simulink model "two_DF_unsplant1"  (Simulink 7.9)
settings: Solver=ode4  SolverMode=SingleTasking  StartTime=0.0  StopTime=120.0  FixedStep=Tm  RelTol=1e-3
InitFcn:
  | initcond
values from neighbouring files (symbols this model uses):
  Delay = 0.5    [initcond.m]    (also in initcond_2DOF_unsplant1.m; initcond_2DOF_unsplant1_copy.m)
  Tm = 0.01    [initcond.m]    (also in initcond_2DOF_unsplant1.m; initcond_2DOF_unsplant1_copy.m)
libraries: fuzblock x3
settings Model: Creator=Ponciano Jorge  LastModifiedBy=cic-pjea  ExtModeTrigMode=oneshot  ExtModeArmWhenConnect=off
settings DataIOCC: LimitDataPoints=off
settings OptimizationCC: BlockReduction=off  BooleanDataType=off  InitFltsAndDblsToZero=on
settings DebuggingCC: SaveWithParameterizedLinksMsg=none  SignalResolutionControl=TryResolveAllWithWarning  SolverPrmCheckMsg=none  MultiTaskDSMMsg=warning  MultiTaskCondExecSysMsg=none  FcnCallInpInsideContextMsg=Use local settings  StrictBusMsg=None
settings HardwareCC: TargetUnknown=on
settings RTWCC: IncludeERTFirstTime=on
settings GRTTargetCC: CombineOutputUpdateFcns=off  GRTInterface=on

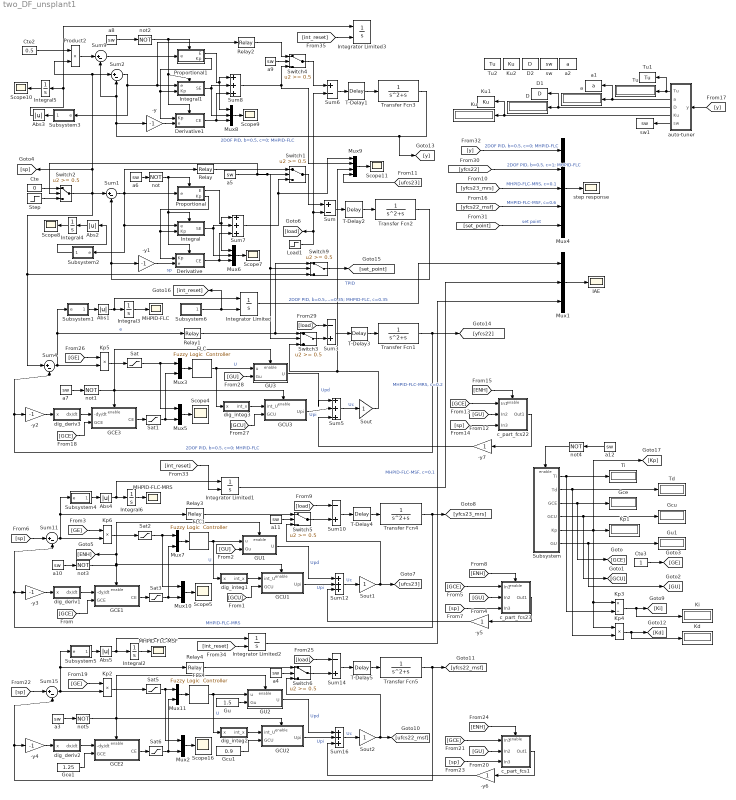
== system two_DF_unsplant1 ==
  -y{,1..4} (5 alike) : Gain  Gain=-1  SaturateOnIntegerOverflow=on  OutDataTypeStr=Inherit: Same as input  ParamDataTypeStr=Inherit: Same as input
  -y5 : Gain  SaturateOnIntegerOverflow=on  OutDataTypeStr=Inherit: Same as input  ParamDataTypeStr=Inherit: Same as input
  -y6 : Gain  SaturateOnIntegerOverflow=on  OutDataTypeStr=Inherit: Same as input  ParamDataTypeStr=Inherit: Same as input
  -y7 : Gain  SaturateOnIntegerOverflow=on  OutDataTypeStr=Inherit: Same as input  ParamDataTypeStr=Inherit: Same as input
  Abs{1..5} (5 alike) : Abs  SaturateOnIntegerOverflow=on
  Cte : Constant  Value=0
  Cte2 : Constant  Value=0.5
  Cte3 : Constant
  D : Display
  D1 : DataStoreWrite  DataStoreName=D
  D2 : DataStoreMemory  DataStoreName=D
  Derivative : Subsystem  TreatAsAtomicUnit=on
  Derivative1 : Subsystem  TreatAsAtomicUnit=on
  FLC : fuzblock/Fuzzy Logic  Controller  fis=stfc22
  FLC1 : fuzblock/Fuzzy Logic  Controller  fis=fcs_unsplan1
  FLC4 : fuzblock/Fuzzy Logic  Controller  fis=stfc22
  GCE1 : Subsystem  TreatAsAtomicUnit=on
  GCE2 : Subsystem  TreatAsAtomicUnit=on
  GCE3 : Subsystem  TreatAsAtomicUnit=on
  GCU1 : Subsystem  TreatAsAtomicUnit=on
  GCU2 : Subsystem  TreatAsAtomicUnit=on
  GCU3 : Subsystem  TreatAsAtomicUnit=on
  GU1 : Subsystem  TreatAsAtomicUnit=on
  GU2 : Subsystem  TreatAsAtomicUnit=on
  GU3 : Subsystem  TreatAsAtomicUnit=on
  Gce : Display
  Gce1 : Constant  Value=1.25
  Gcu : Display
  Gcu1 : Constant  Value=0.9
  Gu : Constant  Value=1.5
  Gu1 : Display
  IAE : Scope
      settings: TickLabels=on  ShowLegends=on  TimeRange=60.03765050579885  YMin=0  YMax=3.5  SaveName=G
  Integral : Subsystem  TreatAsAtomicUnit=on
  Integral1 : Subsystem  TreatAsAtomicUnit=on
  Integral{2..6} (5 alike) : TransferFcn  Denominator=[1 0]
  Integrator Limited{,1..3} (4 alike) : Integrator  ExternalReset=rising  UpperSaturationLimit=1  LowerSaturationLimit=0
  Kd : Display
  Ki : Display
  Kp1 : Display
  Kp2 : Product  SaturateOnIntegerOverflow=on  RndMeth=Zero  InputSameDT=on  OutDataTypeStr=Inherit: Same as first input
  Kp3 : Product  Inputs=*/  SaturateOnIntegerOverflow=on  RndMeth=Zero  InputSameDT=on  OutDataTypeStr=Inherit: Same as first input
  Kp4 : Product  Inputs=**  SaturateOnIntegerOverflow=on  RndMeth=Zero  InputSameDT=on  OutDataTypeStr=Inherit: Same as first input
  Kp5 : Product  SaturateOnIntegerOverflow=on  RndMeth=Zero  InputSameDT=on  OutDataTypeStr=Inherit: Same as first input
  Kp6 : Product  SaturateOnIntegerOverflow=on  RndMeth=Zero  InputSameDT=on  OutDataTypeStr=Inherit: Same as first input
  Ku : Display
  Ku1 : DataStoreWrite  DataStoreName=Ku
  Ku2 : DataStoreMemory  DataStoreName=Ku
  Load1 : Step  Time=92  SampleTime=0
  MHPID-FLC : Scope
      settings: TimeRange=120  YMin=0  YMax=6
  MHPID-FLC-MRS : Scope
      settings: TimeRange=25.06031417248357  YMin=0  YMax=2  SaveName=ScopeData3
  MHPID-FLC-MSF : Scope
      settings: TimeRange=25.04235461740161  YMin=0  YMax=2  SaveName=ScopeData6
  Mux1 : Mux  Inputs=3
  Mux{2..3,5,7,10..11} (6 alike) : Mux  Inputs=2
  Mux4 : Mux  Inputs=5
  Mux6 : Mux  Inputs=3
  Mux8 : Mux  Inputs=3
  Mux9 : Mux
  Product2 : Product  Inputs=**  SaturateOnIntegerOverflow=on  RndMeth=Zero  InputSameDT=on  OutDataTypeStr=Inherit: Same as first input
  Proportional : Subsystem  TreatAsAtomicUnit=on
  Proportional1 : Subsystem  TreatAsAtomicUnit=on
  Relay{,1..4} (5 alike) : Relay  OnOutputValue=0.1  OffOutputValue=-0.1
  Sat{,1..3,5..6} (6 alike) : Saturate  UpperLimit=1  LowerLimit=-1
  Scope{4..5,7..11,16} (8 alike) : Scope
      Scope10 settings: TimeRange=120  YMin=0  YMax=6
      Scope11 settings: TimeRange=50  YMin=-1
      Scope16 settings: TimeRange=40  YMin=-1  YMax=1  SaveName=ScopeData5
      Scope4 settings: TimeRange=50  YMin=-1  YMax=1
      Scope5 settings: TimeRange=40  YMin=-1  YMax=1  SaveName=ScopeData4
      Scope7 settings: TimeRange=50  YMin=-2  YMax=4
      Scope8 settings: TimeRange=120  YMin=0  YMax=7
      Scope9 settings: TimeRange=50  YMin=-2.71141  YMax=4
  Sout : Gain  SaturateOnIntegerOverflow=on  OutDataTypeStr=Inherit: Same as input  ParamDataTypeStr=Inherit: Same as input
  Sout1 : Gain  SaturateOnIntegerOverflow=on  OutDataTypeStr=Inherit: Same as input  ParamDataTypeStr=Inherit: Same as input
  Sout2 : Gain  SaturateOnIntegerOverflow=on  OutDataTypeStr=Inherit: Same as input  ParamDataTypeStr=Inherit: Same as input
  Step : Step  Time=65  SampleTime=0
  Subsystem : Subsystem  TreatAsAtomicUnit=on
  Subsystem1 : Subsystem
  Subsystem2 : Subsystem
  Subsystem3 : Subsystem
  Subsystem4 : Subsystem
  Subsystem5 : Subsystem
  Subsystem6 : Subsystem
  Sum : Sum  Inputs=+-  SaturateOnIntegerOverflow=on  InputSameDT=on  OutDataTypeStr=Inherit: Same as first input
  Sum{1..2,4,9,11,15} (6 alike) : Sum  Inputs=|+-  SaturateOnIntegerOverflow=on  InputSameDT=on  OutDataTypeStr=Inherit: Same as first input
  Sum10 : Sum  Inputs=-+  SaturateOnIntegerOverflow=on  InputSameDT=on  OutDataTypeStr=Inherit: Same as first input
  Sum12 : Sum  Inputs=+++  SaturateOnIntegerOverflow=on  InputSameDT=on  OutDataTypeStr=Inherit: Same as first input
  Sum14 : Sum  Inputs=-+  SaturateOnIntegerOverflow=on  InputSameDT=on  OutDataTypeStr=Inherit: Same as first input
  Sum16 : Sum  Inputs=+++  SaturateOnIntegerOverflow=on  InputSameDT=on  OutDataTypeStr=Inherit: Same as first input
  Sum3 : Sum  Inputs=-+  SaturateOnIntegerOverflow=on  InputSameDT=on  OutDataTypeStr=Inherit: Same as first input
  Sum5 : Sum  Inputs=|+++  SaturateOnIntegerOverflow=on  InputSameDT=on  OutDataTypeStr=Inherit: Same as first input
  Sum6 : Sum  Inputs=+-  SaturateOnIntegerOverflow=on  InputSameDT=on  OutDataTypeStr=Inherit: Same as first input
  Sum7 : Sum  Inputs=|+++  SaturateOnIntegerOverflow=on  InputSameDT=on  OutDataTypeStr=Inherit: Same as first input
  Sum8 : Sum  Inputs=|+++  SaturateOnIntegerOverflow=on  InputSameDT=on  OutDataTypeStr=Inherit: Same as first input
  Switch{1..6,9} (7 alike) : Switch  Threshold=0.5  SaturateOnIntegerOverflow=on  InputSameDT=on
  T-Delay{1..5} (5 alike) : TransportDelay  DelayTime=Delay
  Td : Display
  Ti : Display
  Transfer Fcn{1..5} (5 alike) : TransferFcn  Denominator=[1 1 0]
  Tu : Display
  Tu1 : DataStoreWrite  DataStoreName=Tu
  Tu2 : DataStoreMemory  DataStoreName=Tu  InitialValue=1
  a : Display
  a1 : DataStoreWrite  DataStoreName=a
  a{3..12} (10 alike) : DataStoreRead  DataStoreName=sw  SampleTime=0
  a2 : DataStoreMemory  DataStoreName=a
  auto-tuner : Subsystem
  c_part_fcs1 : Subsystem
  c_part_fcs22 : Subsystem
  c_part_fcs23 : Subsystem
  dig_deriv1 : Subsystem
  dig_deriv2 : Subsystem
  dig_deriv3 : Subsystem
  dig_integ1 : Subsystem
  dig_integ2 : Subsystem
  dig_integ3 : Subsystem
  not{,1..5} (6 alike) : Logic  Operator=NOT
  step response : Scope
      settings: TickLabels=on  ShowLegends=on  TimeRange=60.03765050579885  YMin=-0.2  YMax=1.4  SaveName=G3
  sw : DataStoreMemory  DataStoreName=sw
  sw1 : DataStoreWrite  DataStoreName=sw
  wires:
  T-Delay2/1 -> Transfer Fcn2/1
  Mux3/1 -> FLC/1
  T-Delay3/1 -> Transfer Fcn1/1
  Step/1 -> Switch2/3
  Cte/1 -> Switch2/1
  Transfer Fcn1/1 -> [yfcs22], Sum4/2, -y2/1  "2DOF PID, b=0.5, c=0; MHPID-FLC"
  Sum1/1 -> Proportional/1(e), Integral/1(e), Subsystem2/1(e), Relay/1
  Sum5/1 -> Sout/1  "Uc"
  a6/1 -> not/1
  not/1 -> Proportional/Enable, Integral/Enable, Derivative/Enable
  Proportional/2(Kp) -> Derivative/1(Kp), Integral/2(Kp)
  a7/1 -> not1/1
  Mux5/1 -> Scope4/1
  not1/1 -> GU3/Enable, GCE3/Enable, GCU3/Enable
  Switch2/1 -> Switch9/3, Sum4/1, Sum1/1, Sum2/1, Product2/2, [sp]  "sp"
  Load1/1 -> Sum6/2, Sum/2, [load]
  auto-tuner/1(Tu) -> Tu/1, Tu1/1
  auto-tuner/2(a) -> a/1, a1/1
  auto-tuner/3(D) -> D/1, D1/1
  auto-tuner/4(Ku) -> Ku/1, Ku1/1
  auto-tuner/5(sw) -> sw1/1
  Subsystem1/1(Out1) -> Abs1/1
  Abs1/1 -> Integral3/1, Integrator Limited/1
  Integral3/1 -> MHPID-FLC/1
  Integral4/1 -> Scope8/1
  Abs2/1 -> Integral4/1
  Subsystem2/1(Out1) -> Abs2/1
  Proportional1/2(Kp) -> Derivative1/1(Kp), Integral1/2(Kp)
  a8/1 -> not2/1
  not2/1 -> Proportional1/Enable, Derivative1/Enable, Integral1/Enable
  T-Delay1/1 -> Transfer Fcn3/1
  Product2/1 -> Sum9/1
  Sum2/1 -> Integral1/1(e), Relay2/1, Subsystem3/1(e)
  Sum9/1 -> Proportional1/1(e)
  a5/1 -> Switch1/2, Switch2/2, Switch3/2, Switch9/2
  Mux6/1 -> Scope7/1
  Derivative/1(CE) -> Sum7/3, Mux6/3
  Mux8/1 -> Scope9/1
  Derivative1/1(CE) -> Sum8/3, Mux8/3
  Integral1/1(SE) -> Sum8/2, Mux8/2
  Proportional1/1(E) -> Sum8/1, Mux8/1
  Integral/1(SE) -> Sum7/2, Mux6/2
  Proportional/1(E) -> Sum7/1, Mux6/1
  a9/1 -> Switch4/2
  Relay2/1 -> Switch4/1
  Switch4/1 -> Sum6/1
  Sum4/1 -> Relay1/1, Subsystem1/1(e), Kp5/2  "e"
  Relay/1 -> Switch1/1
  Relay1/1 -> Switch3/1, Switch9/1
  Integral5/1 -> Scope10/1
  Subsystem3/1(Out1) -> Abs3/1
  Abs3/1 -> Integral5/1, Integrator Limited3/1
  Mux9/1 -> Scope11/1
  Sum6/1 -> T-Delay1/1
  Sum/1 -> T-Delay2/1
  Sum3/1 -> T-Delay3/1
  Sum8/1 -> Switch4/3, Mux9/2
  Subsystem/1(Ti) -> Ti/1, Kp3/2
  Subsystem/3(GCE) -> Gce/1, [GCE]
  Subsystem/5(Kp) -> Kp1/1, Kp3/1, Kp4/1, [Kp]
  a12/1 -> not4/1
  not4/1 -> Subsystem/Enable
  Subsystem/2(Td) -> Td/1, Kp4/2
  Subsystem/6(GU) -> Gu1/1, [GU]
  Transfer Fcn3/1 -> Sum2/2, Sum9/2, -y/1, [y]  "2DOF PID, b=0.5, c=0; MHPID-FLC"
  Transfer Fcn2/1 -> Sum1/2, -y1/1  "TPID"
  Switch1/1 -> Sum/1
  Sum7/1 -> Switch1/3, Mux9/1
  Subsystem/4(GCU) -> Gcu/1, [GCU]
  Sat/1 -> Mux3/1, Mux5/1
  Sat1/1 -> Mux3/2, Mux5/2
  GCE3/1(CE) -> Sat1/1
  Switch3/1 -> Sum3/2
  Sout/1 -> Switch3/3, Mux9/3
  dig_deriv3/1(dx/dt) -> GCE3/1(-dy/dt)
  dig_integ3/1(int_x) -> GCU3/1(int_U)
  GCU3/1(Upi) -> Sum5/2  "Upi"
  GU3/1(U) -> Sum5/1  "Upd"
  -y1/1 -> Derivative/2(e)
  -y2/1 -> dig_deriv3/1(x)
  FLC/1 -> dig_integ3/1(x), GU3/1(u)  "U"
  -y/1 -> Derivative1/2(e)
  Cte2/1 -> Product2/1
  Cte3/1 -> [GE]
  [ufcs23] -> Mux9/4
  [GCE] -> c_part_fcs22/1(In1)
  [sp] -> c_part_fcs22/3(In3)
  [GU] -> c_part_fcs22/2(In2)
  [ENH] -> c_part_fcs22/Enable
  Mux7/1 -> FLC1/1
  GCU1/1(Upi) -> Sum12/2  "Upi"
  T-Delay4/1 -> Transfer Fcn4/1
  Sum12/1 -> Sout1/1  "Uc"
  a10/1 -> not3/1
  dig_deriv1/1(dx/dt) -> GCE1/1(-dy/dt)
  Mux10/1 -> Scope5/1
  FLC1/1 -> GU1/1(u), dig_integ1/1(x)  "U"
  GU1/1(U) -> Sum12/1  "Upd"
  Subsystem4/1(Out1) -> Abs4/1
  Abs4/1 -> Integral6/1, Integrator Limited1/1
  Integral6/1 -> MHPID-FLC-MRS/1
  Sum11/1 -> Relay3/1, Subsystem4/1(e), Kp6/2
  Switch5/1 -> Sum10/2
  Sum10/1 -> T-Delay4/1
  GCE1/1(CE) -> Sat3/1
  Sat3/1 -> Mux7/2, Mux10/2
  Kp6/1 -> Sat2/1
  Sat2/1 -> Mux7/1, Mux10/1
  Relay3/1 -> Switch5/1
  a11/1 -> Switch5/2
  Transfer Fcn4/1 -> -y3/1, Sum11/2, [yfcs23_mrs]  "MHPID-FLC-MRS"
  Sout1/1 -> Switch5/3, [ufcs23]
  -y3/1 -> dig_deriv1/1(x)
  [GCE] -> GCE1/2(GCE)
  [GE] -> Kp6/1
  dig_integ1/1(int_x) -> GCU1/1(int_U)
  [GCU] -> GCU1/2(GCU)
  [GU] -> GU1/2(Gu)
  not3/1 -> GCE1/Enable, GCU1/Enable, GU1/Enable, [ENH]
  [GU] -> c_part_fcs23/2(In2)
  [GCE] -> c_part_fcs23/1(In1)
  [sp] -> Sum11/1
  [sp] -> c_part_fcs23/3(In3)
  [ENH] -> c_part_fcs23/Enable
  c_part_fcs23/1(Out1) -> -y5/1
  [load] -> Sum10/1
  Mux11/1 -> FLC4/1
  GCU2/1(Upi) -> Sum16/2  "Upi"
  T-Delay5/1 -> Transfer Fcn5/1
  Sum16/1 -> Sout2/1  "Uc"
  a3/1 -> not5/1
  dig_deriv2/1(dx/dt) -> GCE2/1(-dy/dt)
  Mux2/1 -> Scope16/1
  FLC4/1 -> GU2/1(u), dig_integ2/1(x)  "U"
  GU2/1(U) -> Sum16/1  "Upd"
  Subsystem5/1(Out1) -> Abs5/1
  Abs5/1 -> Integral2/1, Integrator Limited2/1
  Integral2/1 -> MHPID-FLC-MSF/1
  Sum15/1 -> Relay4/1, Subsystem5/1(e), Kp2/2
  Switch6/1 -> Sum14/2
  Sum14/1 -> T-Delay5/1
  GCE2/1(CE) -> Sat6/1
  Sat6/1 -> Mux11/2, Mux2/2
  Kp2/1 -> Sat5/1
  Sat5/1 -> Mux11/1, Mux2/1
  Relay4/1 -> Switch6/1
  a4/1 -> Switch6/2
  Transfer Fcn5/1 -> -y4/1, Sum15/2, [yfcs22_msf]
  Sout2/1 -> Switch6/3, [ufcs22_msf]
  -y4/1 -> dig_deriv2/1(x)
  [GE] -> Kp2/1
  dig_integ2/1(int_x) -> GCU2/1(int_U)
  not5/1 -> GCE2/Enable, GU2/Enable, GCU2/Enable
  [GU] -> c_part_fcs1/2(In2)
  [GCE] -> c_part_fcs1/1(In1)
  [sp] -> Sum15/1
  [sp] -> c_part_fcs1/3(In3)
  [ENH] -> c_part_fcs1/Enable
  [load] -> Sum14/1
  Kp3/1 -> [Ki], Ki/1
  Kp4/1 -> [Kd], Kd/1
  Gu/1 -> GU2/2(Gu)
  Gcu1/1 -> GCU2/2(GCU)
  Gce1/1 -> GCE2/2(GCE)
  c_part_fcs1/1(Out1) -> -y6/1
  -y5/1 -> Sum12/3
  -y6/1 -> Sum16/3
  -y7/1 -> Sum5/3
  Mux1/1 -> IAE/1
  Subsystem6/1(Out1) -> Integrator Limited/2, [int_reset]
  [int_reset] -> Integrator Limited1/2
  Integrator Limited1/1 -> Mux1/2  "MHPID-FLC-MRS, c=0.2"
  [int_reset] -> Integrator Limited2/2
  Integrator Limited2/1 -> Mux1/3  "MHPID-FLC-MSF, c=0.1"
  [y] -> auto-tuner/1(y)
  [GCE] -> GCE3/2(GCE)
  [GE] -> Kp5/1
  Kp5/1 -> Sat/1
  [GCU] -> GCU3/2(GCU)
  [GU] -> GU3/2(Gu)
  [load] -> Sum3/1
  c_part_fcs22/1(Out1) -> -y7/1
  Switch9/1 -> [set_point]
  Mux4/1 -> step response/1
  [int_reset] -> Integrator Limited3/2
  Integrator Limited/1 -> Mux1/1  "2DOF PID, b=0.5, c=0.35; MHPID-FLC, c=0.35"
  [y] -> Mux4/1  "2DOF PID, b=0.5, c=0; MHPID-FLC"
  [yfcs22] -> Mux4/2  "2DOF PID, b=0.5, c=1; MHPID-FLC"
  [yfcs23_mrs] -> Mux4/3  "MHPID-FLC-MRS, c=0.1"
  [yfcs22_msf] -> Mux4/4  "MHPID-FLC-MSF, c=0.6"
  [set_point] -> Mux4/5  "set point"

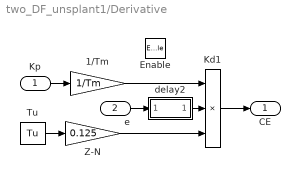
== system two_DF_unsplant1/Derivative ==
  Kp : Inport
  e : Inport  Port=2
  Enable : EnablePort
  1/Tm : Gain  Gain=1/Tm  SaturateOnIntegerOverflow=on  OutDataTypeStr=Inherit: Same as input  ParamDataTypeStr=Inherit: Same as input
  Kd1 : Product  Inputs=3  SaturateOnIntegerOverflow=on  RndMeth=Zero  InputSameDT=on  OutDataTypeStr=Inherit: Same as first input
  Tu : DataStoreRead  DataStoreName=Tu  SampleTime=0
  Z-N : Gain  Gain=0.125  SaturateOnIntegerOverflow=on  OutDataTypeStr=Inherit: Same as input  ParamDataTypeStr=Inherit: Same as input
  delay2 : Subsystem
  CE : Outport
  wires:
  e/1 -> delay2/1(In1)
  Kd1/1 -> CE/1
  Tu/1 -> Z-N/1
  Z-N/1 -> Kd1/3
  Kp/1 -> 1/Tm/1
  1/Tm/1 -> Kd1/1
  delay2/1(Out1) -> Kd1/2

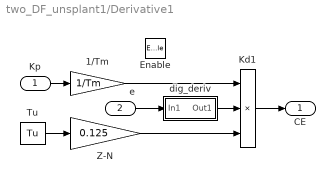
== system two_DF_unsplant1/Derivative1 ==
  Kp : Inport
  e : Inport  Port=2
  Enable : EnablePort
  1/Tm : Gain  Gain=1/Tm  SaturateOnIntegerOverflow=on  OutDataTypeStr=Inherit: Same as input  ParamDataTypeStr=Inherit: Same as input
  Kd1 : Product  Inputs=3  SaturateOnIntegerOverflow=on  RndMeth=Zero  InputSameDT=on  OutDataTypeStr=Inherit: Same as first input
  Tu : DataStoreRead  DataStoreName=Tu  SampleTime=0
  Z-N : Gain  Gain=0.125  SaturateOnIntegerOverflow=on  OutDataTypeStr=Inherit: Same as input  ParamDataTypeStr=Inherit: Same as input
  dig_deriv : Subsystem
  CE : Outport
  wires:
  e/1 -> dig_deriv/1(In1)
  Kd1/1 -> CE/1
  Tu/1 -> Z-N/1
  Z-N/1 -> Kd1/3
  Kp/1 -> 1/Tm/1
  1/Tm/1 -> Kd1/1
  dig_deriv/1(Out1) -> Kd1/2

== system two_DF_unsplant1/GCE1 ==
  -dy/dt : Inport
  GCE : Inport  Port=2
  Enable : EnablePort
  Kp6 : Product  SaturateOnIntegerOverflow=on  RndMeth=Zero  InputSameDT=on  OutDataTypeStr=Inherit: Same as first input
  CE : Outport
  wires:
  Kp6/1 -> CE/1
  GCE/1 -> Kp6/1
  -dy/dt/1 -> Kp6/2

== system two_DF_unsplant1/GCE2 ==
  -dy/dt : Inport
  GCE : Inport  Port=2
  Enable : EnablePort
  Kp6 : Product  SaturateOnIntegerOverflow=on  RndMeth=Zero  InputSameDT=on  OutDataTypeStr=Inherit: Same as first input
  CE : Outport
  wires:
  Kp6/1 -> CE/1
  GCE/1 -> Kp6/1
  -dy/dt/1 -> Kp6/2

== system two_DF_unsplant1/GCE3 ==
  -dy/dt : Inport
  GCE : Inport  Port=2
  Enable : EnablePort
  Kp6 : Product  SaturateOnIntegerOverflow=on  RndMeth=Zero  InputSameDT=on  OutDataTypeStr=Inherit: Same as first input
  CE : Outport
  wires:
  Kp6/1 -> CE/1
  GCE/1 -> Kp6/1
  -dy/dt/1 -> Kp6/2

== system two_DF_unsplant1/GCU1 ==
  int_U : Inport
  GCU : Inport  Port=2
  Enable : EnablePort
  Kp5 : Product  SaturateOnIntegerOverflow=on  RndMeth=Zero  InputSameDT=on  OutDataTypeStr=Inherit: Same as first input
  Upi : Outport
  wires:
  Kp5/1 -> Upi/1
  int_U/1 -> Kp5/1
  GCU/1 -> Kp5/2

== system two_DF_unsplant1/GCU2 ==
  int_U : Inport
  GCU : Inport  Port=2
  Enable : EnablePort
  Kp5 : Product  SaturateOnIntegerOverflow=on  RndMeth=Zero  InputSameDT=on  OutDataTypeStr=Inherit: Same as first input
  Upi : Outport
  wires:
  Kp5/1 -> Upi/1
  int_U/1 -> Kp5/1
  GCU/1 -> Kp5/2

== system two_DF_unsplant1/GCU3 ==
  int_U : Inport
  GCU : Inport  Port=2
  Enable : EnablePort
  Kp5 : Product  SaturateOnIntegerOverflow=on  RndMeth=Zero  InputSameDT=on  OutDataTypeStr=Inherit: Same as first input
  Upi : Outport
  wires:
  Kp5/1 -> Upi/1
  int_U/1 -> Kp5/1
  GCU/1 -> Kp5/2

== system two_DF_unsplant1/GU1 ==
  u : Inport
  Gu : Inport  Port=2
  Enable : EnablePort
  Kp7 : Product  SaturateOnIntegerOverflow=on  RndMeth=Zero  InputSameDT=on  OutDataTypeStr=Inherit: Same as first input
  U : Outport
  wires:
  Kp7/1 -> U/1
  u/1 -> Kp7/1
  Gu/1 -> Kp7/2

== system two_DF_unsplant1/GU2 ==
  u : Inport
  Gu : Inport  Port=2
  Enable : EnablePort
  Kp7 : Product  SaturateOnIntegerOverflow=on  RndMeth=Zero  InputSameDT=on  OutDataTypeStr=Inherit: Same as first input
  U : Outport
  wires:
  Kp7/1 -> U/1
  u/1 -> Kp7/1
  Gu/1 -> Kp7/2

== system two_DF_unsplant1/GU3 ==
  u : Inport
  Gu : Inport  Port=2
  Enable : EnablePort
  Kp7 : Product  SaturateOnIntegerOverflow=on  RndMeth=Zero  InputSameDT=on  OutDataTypeStr=Inherit: Same as first input
  U : Outport
  wires:
  Kp7/1 -> U/1
  u/1 -> Kp7/1
  Gu/1 -> Kp7/2

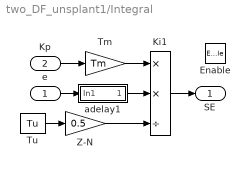
== system two_DF_unsplant1/Integral ==
  e : Inport
  Kp : Inport  Port=2
  Enable : EnablePort
  Ki1 : Product  Inputs=**/  SaturateOnIntegerOverflow=on  RndMeth=Zero  InputSameDT=on  OutDataTypeStr=Inherit: Same as first input
  Tm : Gain  Gain=Tm  SaturateOnIntegerOverflow=on  OutDataTypeStr=Inherit: Same as input  ParamDataTypeStr=Inherit: Same as input
  Tu : DataStoreRead  DataStoreName=Tu  SampleTime=0
  Z-N : Gain  Gain=0.5  SaturateOnIntegerOverflow=on  OutDataTypeStr=Inherit: Same as input  ParamDataTypeStr=Inherit: Same as input
  adelay1 : Subsystem
  SE : Outport
  wires:
  adelay1/1(Out1) -> Ki1/2
  Z-N/1 -> Ki1/3
  e/1 -> adelay1/1(In1)
  Ki1/1 -> SE/1
  Tu/1 -> Z-N/1
  Kp/1 -> Tm/1
  Tm/1 -> Ki1/1

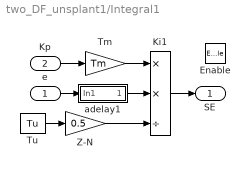
== system two_DF_unsplant1/Integral1 ==
  e : Inport
  Kp : Inport  Port=2
  Enable : EnablePort
  Ki1 : Product  Inputs=**/  SaturateOnIntegerOverflow=on  RndMeth=Zero  InputSameDT=on  OutDataTypeStr=Inherit: Same as first input
  Tm : Gain  Gain=Tm  SaturateOnIntegerOverflow=on  OutDataTypeStr=Inherit: Same as input  ParamDataTypeStr=Inherit: Same as input
  Tu : DataStoreRead  DataStoreName=Tu  SampleTime=0
  Z-N : Gain  Gain=0.5  SaturateOnIntegerOverflow=on  OutDataTypeStr=Inherit: Same as input  ParamDataTypeStr=Inherit: Same as input
  adelay1 : Subsystem
  SE : Outport
  wires:
  adelay1/1(Out1) -> Ki1/2
  Z-N/1 -> Ki1/3
  e/1 -> adelay1/1(In1)
  Ki1/1 -> SE/1
  Tu/1 -> Z-N/1
  Kp/1 -> Tm/1
  Tm/1 -> Ki1/1

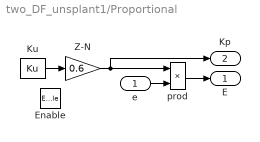
== system two_DF_unsplant1/Proportional ==
  e : Inport
  Enable : EnablePort
  Ku : DataStoreRead  DataStoreName=Ku  SampleTime=0
  Z-N : Gain  Gain=0.6  SaturateOnIntegerOverflow=on  OutDataTypeStr=Inherit: Same as input  ParamDataTypeStr=Inherit: Same as input
  prod : Product  SaturateOnIntegerOverflow=on  RndMeth=Zero  InputSameDT=on  OutDataTypeStr=Inherit: Same as first input
  E : Outport
  Kp : Outport  Port=2
  wires:
  Ku/1 -> Z-N/1
  prod/1 -> E/1
  e/1 -> prod/2
  Z-N/1 -> Kp/1, prod/1

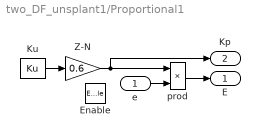
== system two_DF_unsplant1/Proportional1 ==
  e : Inport
  Enable : EnablePort
  Ku : DataStoreRead  DataStoreName=Ku  SampleTime=0
  Z-N : Gain  Gain=0.6  SaturateOnIntegerOverflow=on  OutDataTypeStr=Inherit: Same as input  ParamDataTypeStr=Inherit: Same as input
  prod : Product  SaturateOnIntegerOverflow=on  RndMeth=Zero  InputSameDT=on  OutDataTypeStr=Inherit: Same as first input
  E : Outport
  Kp : Outport  Port=2
  wires:
  prod/1 -> E/1
  e/1 -> prod/2
  Z-N/1 -> prod/1, Kp/1
  Ku/1 -> Z-N/1

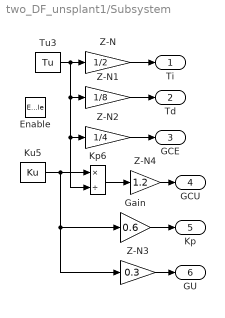
== system two_DF_unsplant1/Subsystem ==
  Enable : EnablePort
  Gain : Gain  Gain=0.6  SaturateOnIntegerOverflow=on  OutDataTypeStr=Inherit: Same as input  ParamDataTypeStr=Inherit: Same as input
  Kp6 : Product  Inputs=*/  SaturateOnIntegerOverflow=on  RndMeth=Zero  InputSameDT=on  OutDataTypeStr=Inherit: Same as first input
  Ku5 : DataStoreRead  DataStoreName=Ku  SampleTime=0
  Tu3 : DataStoreRead  DataStoreName=Tu  SampleTime=0
  Z-N : Gain  Gain=1/2  SaturateOnIntegerOverflow=on  OutDataTypeStr=Inherit: Same as input  ParamDataTypeStr=Inherit: Same as input
  Z-N1 : Gain  Gain=1/8  SaturateOnIntegerOverflow=on  OutDataTypeStr=Inherit: Same as input  ParamDataTypeStr=Inherit: Same as input
  Z-N2 : Gain  Gain=1/4  SaturateOnIntegerOverflow=on  OutDataTypeStr=Inherit: Same as input  ParamDataTypeStr=Inherit: Same as input
  Z-N3 : Gain  Gain=0.3  SaturateOnIntegerOverflow=on  OutDataTypeStr=Inherit: Same as input  ParamDataTypeStr=Inherit: Same as input
  Z-N4 : Gain  Gain=1.2  SaturateOnIntegerOverflow=on  OutDataTypeStr=Inherit: Same as input  ParamDataTypeStr=Inherit: Same as input
  Ti : Outport
  Td : Outport  Port=2
  GCE : Outport  Port=3
  GCU : Outport  Port=4
  Kp : Outport  Port=5
  GU : Outport  Port=6
  wires:
  Tu3/1 -> Z-N/1, Z-N1/1, Z-N2/1, Kp6/2
  Kp6/1 -> Z-N4/1
  Z-N/1 -> Ti/1
  Z-N1/1 -> Td/1
  Z-N2/1 -> GCE/1
  Z-N4/1 -> GCU/1
  Z-N3/1 -> GU/1
  Gain/1 -> Kp/1
  Ku5/1 -> Kp6/1, Gain/1, Z-N3/1

== system two_DF_unsplant1/Subsystem1 ==
  e : Inport
  Clock1 : Clock
  Equal3 : RelationalOperator  Operator=<  InputSameDT=on
  Switch4 : Switch  Threshold=0.5  SaturateOnIntegerOverflow=on  InputSameDT=on
  zero : Constant  Value=0
  zero1 : Constant  Value=60
  Out1 : Outport
  wires:
  Clock1/1 -> Equal3/1
  zero1/1 -> Equal3/2
  Switch4/1 -> Out1/1
  e/1 -> Switch4/3
  zero/1 -> Switch4/1
  Equal3/1 -> Switch4/2

== system two_DF_unsplant1/Subsystem2 ==
  e : Inport
  Clock1 : Clock
  Equal3 : RelationalOperator  Operator=<  InputSameDT=on
  Switch4 : Switch  Threshold=0.5  SaturateOnIntegerOverflow=on  InputSameDT=on
  zero : Constant  Value=0
  zero1 : Constant  Value=60
  Out1 : Outport
  wires:
  Clock1/1 -> Equal3/1
  zero1/1 -> Equal3/2
  Switch4/1 -> Out1/1
  e/1 -> Switch4/3
  zero/1 -> Switch4/1
  Equal3/1 -> Switch4/2

== system two_DF_unsplant1/Subsystem3 ==
  e : Inport
  Clock1 : Clock
  Equal3 : RelationalOperator  Operator=<  InputSameDT=on
  Switch4 : Switch  Threshold=0.5  SaturateOnIntegerOverflow=on  InputSameDT=on
  zero : Constant  Value=0
  zero1 : Constant  Value=60
  Out1 : Outport
  wires:
  Clock1/1 -> Equal3/1
  zero1/1 -> Equal3/2
  Switch4/1 -> Out1/1
  e/1 -> Switch4/3
  zero/1 -> Switch4/1
  Equal3/1 -> Switch4/2

== system two_DF_unsplant1/Subsystem4 ==
  e : Inport
  Clock1 : Clock
  Equal3 : RelationalOperator  Operator=<  InputSameDT=on
  Switch4 : Switch  Threshold=0.5  SaturateOnIntegerOverflow=on  InputSameDT=on
  zero : Constant  Value=0
  zero1 : Constant  Value=60
  Out1 : Outport
  wires:
  Clock1/1 -> Equal3/1
  zero1/1 -> Equal3/2
  Switch4/1 -> Out1/1
  e/1 -> Switch4/3
  zero/1 -> Switch4/1
  Equal3/1 -> Switch4/2

== system two_DF_unsplant1/Subsystem5 ==
  e : Inport
  Clock1 : Clock
  Equal3 : RelationalOperator  Operator=<  InputSameDT=on
  Switch4 : Switch  Threshold=0.5  SaturateOnIntegerOverflow=on  InputSameDT=on
  zero : Constant  Value=0
  zero1 : Constant  Value=60
  Out1 : Outport
  wires:
  Clock1/1 -> Equal3/1
  zero1/1 -> Equal3/2
  Switch4/1 -> Out1/1
  e/1 -> Switch4/3
  zero/1 -> Switch4/1
  Equal3/1 -> Switch4/2

== system two_DF_unsplant1/Subsystem6 ==
  Clock1 : Clock
  Equal3 : RelationalOperator  Operator===  InputSameDT=on
  zero1 : Constant  Value=90
  Out1 : Outport
  wires:
  Clock1/1 -> Equal3/1
  zero1/1 -> Equal3/2
  Equal3/1 -> Out1/1

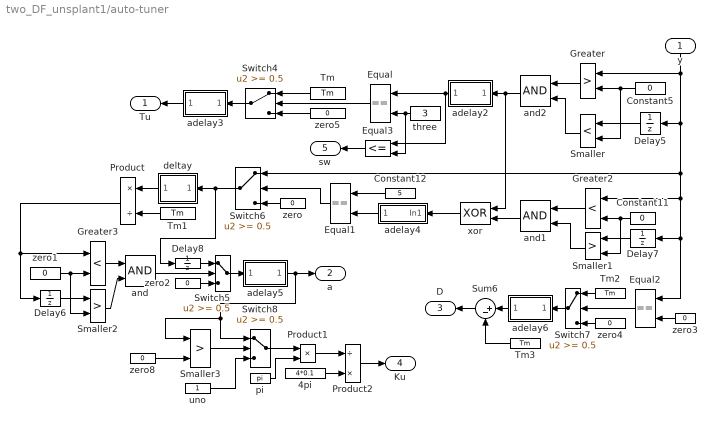
== system two_DF_unsplant1/auto-tuner ==
  y : Inport
  4pi : Constant  Value=4*0.1
  Constant11 : Constant  Value=0
  Constant12 : Constant  Value=5
  Constant5 : Constant  Value=0
  Delay{5..8} (4 alike) : UnitDelay  SampleTime=Tm
  Equal : RelationalOperator  Operator===  InputSameDT=on
  Equal1 : RelationalOperator  Operator===  InputSameDT=on
  Equal2 : RelationalOperator  Operator===  InputSameDT=on
  Equal3 : RelationalOperator  Operator=<=  InputSameDT=on
  Greater : RelationalOperator  Operator=>  InputSameDT=on
  Greater2 : RelationalOperator  Operator=<  InputSameDT=on
  Greater3 : RelationalOperator  Operator=<  InputSameDT=on
  Product : Product  Inputs=*/  SaturateOnIntegerOverflow=on  RndMeth=Zero  InputSameDT=on  OutDataTypeStr=Inherit: Same as first input
  Product1 : Product  SaturateOnIntegerOverflow=on  RndMeth=Zero  InputSameDT=on  OutDataTypeStr=Inherit: Same as first input
  Product2 : Product  Inputs=/*  SaturateOnIntegerOverflow=on  RndMeth=Zero  InputSameDT=on  OutDataTypeStr=Inherit: Same as first input
  Smaller : RelationalOperator  Operator=<  InputSameDT=on
  Smaller1 : RelationalOperator  Operator=>  InputSameDT=on
  Smaller2 : RelationalOperator  Operator=>  InputSameDT=on
  Smaller3 : RelationalOperator  Operator=>  InputSameDT=on
  Sum6 : Sum  Inputs=|+-  SaturateOnIntegerOverflow=on  InputSameDT=on  OutDataTypeStr=Inherit: Same as first input
  Switch{4..8} (5 alike) : Switch  Threshold=0.5  SaturateOnIntegerOverflow=on  InputSameDT=on
  Tm{,1..3} (4 alike) : Constant  Value=Tm
  adelay2 : Subsystem
  adelay3 : Subsystem
  adelay4 : Subsystem
  adelay5 : Subsystem
  adelay6 : Subsystem
  and : Logic
  and1 : Logic
  and2 : Logic
  deltay : Subsystem
  pi : Constant  Value=pi
  three : Constant  Value=3
  uno : Constant
  xor : Logic  Operator=XOR
  zero{,1..5,8} (7 alike) : Constant  Value=0
  Tu : Outport
  a : Outport  Port=2
  D : Outport  Port=3
  Ku : Outport  Port=4
  sw : Outport  Port=5
  wires:
  y/1 -> Greater/1, Delay5/1, Greater2/1, Delay7/1, Equal2/1, Switch6/1
  Delay5/1 -> Smaller/1
  Greater/1 -> and2/1
  Smaller/1 -> and2/2
  Constant5/1 -> Greater/2, Smaller/2
  zero5/1 -> Switch4/3
  Switch4/1 -> adelay3/1(In1)
  zero/1 -> Switch6/3
  Tm/1 -> Switch4/1
  Delay7/1 -> Smaller1/1
  Greater2/1 -> and1/1
  Smaller1/1 -> and1/2
  Constant11/1 -> Greater2/2, Smaller1/2
  Constant12/1 -> Equal1/1
  deltay/1(Out1) -> Product/1
  Tm1/1 -> Product/2
  Delay6/1 -> Smaller2/1
  Greater3/1 -> and/1
  Smaller2/1 -> and/2
  zero1/1 -> Greater3/2, Smaller2/2
  Delay8/1 -> Switch5/1
  Switch6/1 -> deltay/1(In1), Delay8/1
  and/1 -> Switch5/2
  Product/1 -> Greater3/1, Delay6/1
  zero2/1 -> Switch5/3
  Equal1/1 -> Switch6/2
  Switch5/1 -> adelay5/1(In1)
  zero3/1 -> Equal2/2
  Equal2/1 -> Switch7/2
  Tm2/1 -> Switch7/1
  zero4/1 -> Switch7/3
  Tm3/1 -> Sum6/2
  adelay6/1(Out1) -> Sum6/1
  Switch7/1 -> adelay6/1(In1)
  zero8/1 -> Smaller3/2
  Smaller3/1 -> Switch8/2
  uno/1 -> Switch8/3
  Product1/1 -> Product2/1
  4pi/1 -> Product2/2
  pi/1 -> Product1/2
  Switch8/1 -> Product1/1
  three/1 -> Equal/2, Equal3/2
  adelay2/1(Out1) -> Equal/1, Equal3/1
  and2/1 -> adelay2/1(In1), xor/1
  xor/1 -> adelay4/1(In1)
  adelay3/1(Out1) -> Tu/1
  adelay5/1(Out1) -> a/1, Switch8/1, Smaller3/1
  Sum6/1 -> D/1
  Product2/1 -> Ku/1
  Equal3/1 -> sw/1
  Equal/1 -> Switch4/2
  adelay4/1(Out1) -> Equal1/2
  and1/1 -> xor/2

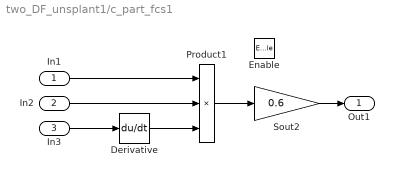
== system two_DF_unsplant1/c_part_fcs1 ==
  In1 : Inport
  In2 : Inport  Port=2
  In3 : Inport  Port=3
  Enable : EnablePort
  Derivative : Derivative
  Product1 : Product  Inputs=***  SaturateOnIntegerOverflow=on  RndMeth=Zero  InputSameDT=on  OutDataTypeStr=Inherit: Same as first input
  Sout2 : Gain  Gain=0.6  SaturateOnIntegerOverflow=on  OutDataTypeStr=Inherit: Same as input  ParamDataTypeStr=Inherit: Same as input
  Out1 : Outport
  wires:
  Product1/1 -> Sout2/1
  In1/1 -> Product1/1
  In2/1 -> Product1/2
  Sout2/1 -> Out1/1
  In3/1 -> Derivative/1
  Derivative/1 -> Product1/3

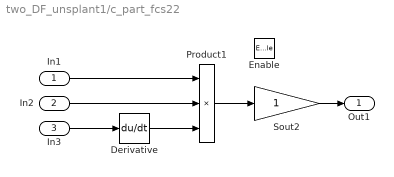
== system two_DF_unsplant1/c_part_fcs22 ==
  In1 : Inport
  In2 : Inport  Port=2
  In3 : Inport  Port=3
  Enable : EnablePort
  Derivative : Derivative
  Product1 : Product  Inputs=***  SaturateOnIntegerOverflow=on  RndMeth=Zero  InputSameDT=on  OutDataTypeStr=Inherit: Same as first input
  Sout2 : Gain  SaturateOnIntegerOverflow=on  OutDataTypeStr=Inherit: Same as input  ParamDataTypeStr=Inherit: Same as input
  Out1 : Outport
  wires:
  Product1/1 -> Sout2/1
  In1/1 -> Product1/1
  In2/1 -> Product1/2
  Sout2/1 -> Out1/1
  In3/1 -> Derivative/1
  Derivative/1 -> Product1/3

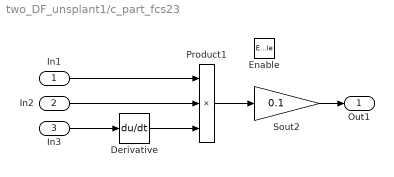
== system two_DF_unsplant1/c_part_fcs23 ==
  In1 : Inport
  In2 : Inport  Port=2
  In3 : Inport  Port=3
  Enable : EnablePort
  Derivative : Derivative
  Product1 : Product  Inputs=***  SaturateOnIntegerOverflow=on  RndMeth=Zero  InputSameDT=on  OutDataTypeStr=Inherit: Same as first input
  Sout2 : Gain  Gain=0.1  SaturateOnIntegerOverflow=on  OutDataTypeStr=Inherit: Same as input  ParamDataTypeStr=Inherit: Same as input
  Out1 : Outport
  wires:
  Product1/1 -> Sout2/1
  In1/1 -> Product1/1
  In2/1 -> Product1/2
  Sout2/1 -> Out1/1
  In3/1 -> Derivative/1
  Derivative/1 -> Product1/3

== system two_DF_unsplant1/dig_deriv1 ==
  x : Inport
  1/Tm : Gain  Gain=1/Tm  SaturateOnIntegerOverflow=on  OutDataTypeStr=Inherit: Same as input  ParamDataTypeStr=Inherit: Same as input
  Sum9 : Sum  Inputs=|+-  SaturateOnIntegerOverflow=on  InputSameDT=on  OutDataTypeStr=Inherit: Same as first input
  Unit Delay5 : UnitDelay  SampleTime=Tm
  dx/dt : Outport
  wires:
  x/1 -> Sum9/1, Unit Delay5/1
  Unit Delay5/1 -> Sum9/2
  Sum9/1 -> 1/Tm/1
  1/Tm/1 -> dx/dt/1

== system two_DF_unsplant1/dig_deriv2 ==
  x : Inport
  1/Tm : Gain  Gain=1/Tm  SaturateOnIntegerOverflow=on  OutDataTypeStr=Inherit: Same as input  ParamDataTypeStr=Inherit: Same as input
  Sum9 : Sum  Inputs=|+-  SaturateOnIntegerOverflow=on  InputSameDT=on  OutDataTypeStr=Inherit: Same as first input
  Unit Delay5 : UnitDelay  SampleTime=Tm
  dx/dt : Outport
  wires:
  x/1 -> Sum9/1, Unit Delay5/1
  Unit Delay5/1 -> Sum9/2
  Sum9/1 -> 1/Tm/1
  1/Tm/1 -> dx/dt/1

== system two_DF_unsplant1/dig_deriv3 ==
  x : Inport
  1/Tm : Gain  Gain=1/Tm  SaturateOnIntegerOverflow=on  OutDataTypeStr=Inherit: Same as input  ParamDataTypeStr=Inherit: Same as input
  Sum9 : Sum  Inputs=|+-  SaturateOnIntegerOverflow=on  InputSameDT=on  OutDataTypeStr=Inherit: Same as first input
  Unit Delay5 : UnitDelay  SampleTime=Tm
  dx/dt : Outport
  wires:
  x/1 -> Sum9/1, Unit Delay5/1
  Unit Delay5/1 -> Sum9/2
  Sum9/1 -> 1/Tm/1
  1/Tm/1 -> dx/dt/1

== system two_DF_unsplant1/dig_integ1 ==
  x : Inport
  Sum9 : Sum  Inputs=|++  SaturateOnIntegerOverflow=on  InputSameDT=on  OutDataTypeStr=Inherit: Same as first input
  Tm : Gain  Gain=Tm  SaturateOnIntegerOverflow=on  OutDataTypeStr=Inherit: Same as input  ParamDataTypeStr=Inherit: Same as input
  Unit Delay6 : UnitDelay  SampleTime=Tm
  int_x : Outport
  wires:
  Sum9/1 -> Unit Delay6/1, Tm/1
  Unit Delay6/1 -> Sum9/2
  x/1 -> Sum9/1
  Tm/1 -> int_x/1

== system two_DF_unsplant1/dig_integ2 ==
  x : Inport
  Sum9 : Sum  Inputs=|++  SaturateOnIntegerOverflow=on  InputSameDT=on  OutDataTypeStr=Inherit: Same as first input
  Tm : Gain  Gain=Tm  SaturateOnIntegerOverflow=on  OutDataTypeStr=Inherit: Same as input  ParamDataTypeStr=Inherit: Same as input
  Unit Delay6 : UnitDelay  SampleTime=Tm
  int_x : Outport
  wires:
  Sum9/1 -> Unit Delay6/1, Tm/1
  Unit Delay6/1 -> Sum9/2
  x/1 -> Sum9/1
  Tm/1 -> int_x/1

== system two_DF_unsplant1/dig_integ3 ==
  x : Inport
  Sum9 : Sum  Inputs=|++  SaturateOnIntegerOverflow=on  InputSameDT=on  OutDataTypeStr=Inherit: Same as first input
  Tm : Gain  Gain=Tm  SaturateOnIntegerOverflow=on  OutDataTypeStr=Inherit: Same as input  ParamDataTypeStr=Inherit: Same as input
  Unit Delay6 : UnitDelay  SampleTime=Tm
  int_x : Outport
  wires:
  Sum9/1 -> Unit Delay6/1, Tm/1
  Unit Delay6/1 -> Sum9/2
  x/1 -> Sum9/1
  Tm/1 -> int_x/1

== system two_DF_unsplant1/Derivative/delay2 ==
  In1 : Inport
  Sum9 : Sum  Inputs=|+-  SaturateOnIntegerOverflow=on  InputSameDT=on  OutDataTypeStr=Inherit: Same as first input
  Unit Delay5 : UnitDelay  SampleTime=Tm
  Out1 : Outport
  wires:
  Sum9/1 -> Out1/1
  In1/1 -> Sum9/1, Unit Delay5/1
  Unit Delay5/1 -> Sum9/2

== system two_DF_unsplant1/Derivative1/dig_deriv ==
  In1 : Inport
  Sum9 : Sum  Inputs=|+-  SaturateOnIntegerOverflow=on  InputSameDT=on  OutDataTypeStr=Inherit: Same as first input
  Unit Delay5 : UnitDelay  SampleTime=Tm
  Out1 : Outport
  wires:
  Sum9/1 -> Out1/1
  In1/1 -> Sum9/1, Unit Delay5/1
  Unit Delay5/1 -> Sum9/2

== system two_DF_unsplant1/Integral/adelay1 ==
  In1 : Inport
  Sum9 : Sum  Inputs=|++  SaturateOnIntegerOverflow=on  InputSameDT=on  OutDataTypeStr=Inherit: Same as first input
  Unit Delay6 : UnitDelay  SampleTime=Tm
  Out1 : Outport
  wires:
  In1/1 -> Sum9/1
  Unit Delay6/1 -> Sum9/2
  Sum9/1 -> Out1/1, Unit Delay6/1

== system two_DF_unsplant1/Integral1/adelay1 ==
  In1 : Inport
  Sum9 : Sum  Inputs=|++  SaturateOnIntegerOverflow=on  InputSameDT=on  OutDataTypeStr=Inherit: Same as first input
  Unit Delay6 : UnitDelay  SampleTime=Tm
  Out1 : Outport
  wires:
  In1/1 -> Sum9/1
  Unit Delay6/1 -> Sum9/2
  Sum9/1 -> Out1/1, Unit Delay6/1

== system two_DF_unsplant1/auto-tuner/adelay2 ==
  In1 : Inport
  Sum9 : Sum  Inputs=|++  SaturateOnIntegerOverflow=on  InputSameDT=on  OutDataTypeStr=Inherit: Same as first input
  Unit Delay6 : UnitDelay  SampleTime=Tm
  Out1 : Outport
  wires:
  In1/1 -> Sum9/1
  Unit Delay6/1 -> Sum9/2
  Sum9/1 -> Out1/1, Unit Delay6/1

== system two_DF_unsplant1/auto-tuner/adelay3 ==
  In1 : Inport
  Sum9 : Sum  Inputs=|++  SaturateOnIntegerOverflow=on  InputSameDT=on  OutDataTypeStr=Inherit: Same as first input
  Unit Delay6 : UnitDelay  SampleTime=Tm
  Out1 : Outport
  wires:
  In1/1 -> Sum9/1
  Unit Delay6/1 -> Sum9/2
  Sum9/1 -> Out1/1, Unit Delay6/1

== system two_DF_unsplant1/auto-tuner/adelay4 ==
  In1 : Inport
  Sum9 : Sum  Inputs=|++  SaturateOnIntegerOverflow=on  InputSameDT=on  OutDataTypeStr=Inherit: Same as first input
  Unit Delay6 : UnitDelay  SampleTime=Tm
  Out1 : Outport
  wires:
  In1/1 -> Sum9/1
  Unit Delay6/1 -> Sum9/2
  Sum9/1 -> Out1/1, Unit Delay6/1

== system two_DF_unsplant1/auto-tuner/adelay5 ==
  In1 : Inport
  Sum9 : Sum  Inputs=|++  SaturateOnIntegerOverflow=on  InputSameDT=on  OutDataTypeStr=Inherit: Same as first input
  Unit Delay6 : UnitDelay  SampleTime=Tm
  Out1 : Outport
  wires:
  In1/1 -> Sum9/1
  Unit Delay6/1 -> Sum9/2
  Sum9/1 -> Out1/1, Unit Delay6/1

== system two_DF_unsplant1/auto-tuner/adelay6 ==
  In1 : Inport
  Sum9 : Sum  Inputs=|++  SaturateOnIntegerOverflow=on  InputSameDT=on  OutDataTypeStr=Inherit: Same as first input
  Unit Delay6 : UnitDelay  SampleTime=Tm
  Out1 : Outport
  wires:
  In1/1 -> Sum9/1
  Unit Delay6/1 -> Sum9/2
  Sum9/1 -> Out1/1, Unit Delay6/1

== system two_DF_unsplant1/auto-tuner/deltay ==
  In1 : Inport
  Sum9 : Sum  Inputs=|+-  SaturateOnIntegerOverflow=on  InputSameDT=on  OutDataTypeStr=Inherit: Same as first input
  Unit Delay5 : UnitDelay  SampleTime=Tm
  Out1 : Outport
  wires:
  In1/1 -> Sum9/1, Unit Delay5/1
  Unit Delay5/1 -> Sum9/2
  Sum9/1 -> Out1/1
